simulink model "task_3"  (R2024a)
settings: Solver=VariableStepAuto  StartTime=0.0  StopTime=10.0  RelTol=1e-3
settings Model: Creator=alexe  LastModifiedBy=alexe

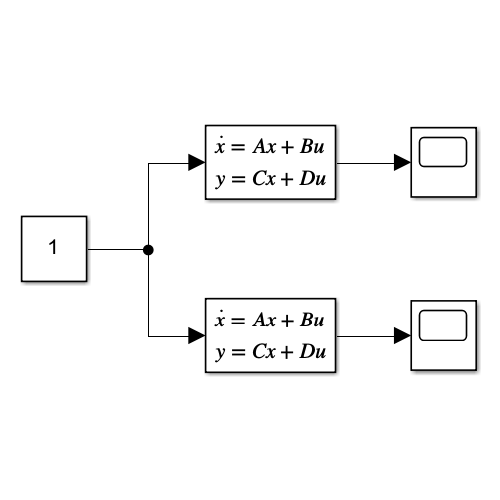
[thumbnail: Simulink's stored preview of the top-level diagram]
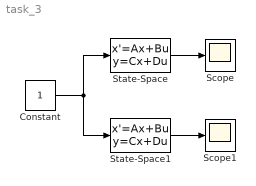
== system task_3 ==
  Constant : Constant
  Scope : Scope
  Scope1 : Scope
  State-Space : StateSpace  A=[0.5 1; -15 -3]  B=[0;1]  C=[5 1]  D=0  InitialCondition=0
  State-Space1 : StateSpace  A=[3 0.25; -120 -5.5]  B=[0;2]  C=[15 0.5]  D=0  InitialCondition=0
  wires:
  Constant/1 -> State-Space1/1, State-Space/1
  State-Space/1 -> Scope/1
  State-Space1/1 -> Scope1/1
